simulink model "example9"  (Simulink 6.0)
settings: Solver=ode45  StartTime=0.0  StopTime=100  RelTol=1e-4
undefined symbols (not defined in the file or in its folder): adaptive_passivity, forward_kin_2link, hgoder_2link, parameter_adapt, stateder, Z0, Zhat0
libraries: simulink x1
settings Model: Creator=rhanz  LastModifiedBy=rhanz  ExtModeAutoUpdateStatusClock=off
settings DataIOCC: Refine=2
settings OptimizationCC: InlineInvariantSignals=off

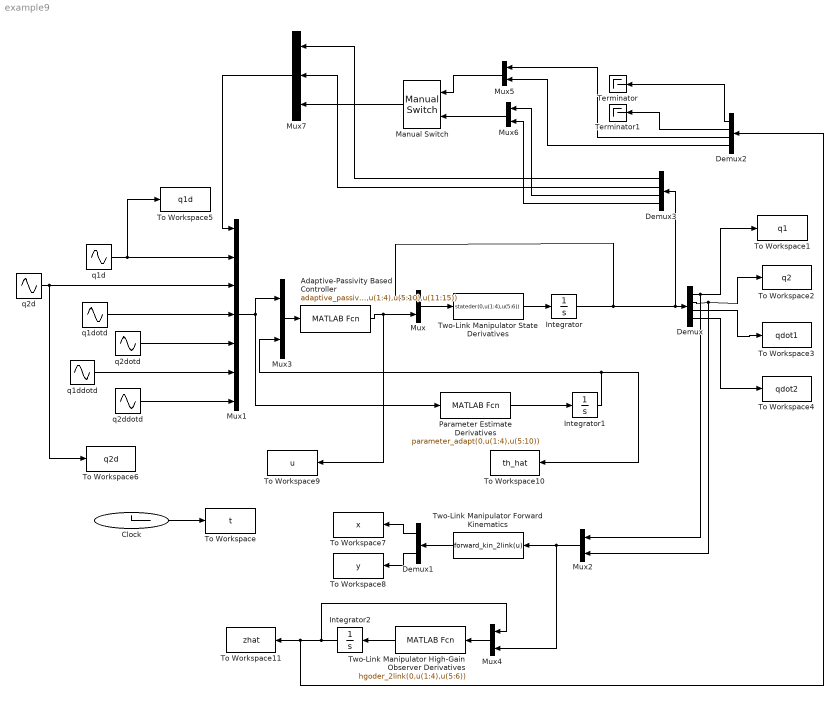
== system example9 ==
  Adaptive-Passivity Based Controller : MATLABFcn  MATLABFcn=adaptive_passivity(0,u(1:4),u(5:10),u(11:15))  OutputDimensions=2
  Clock : Clock
      settings: Decimation=10
  Demux : Demux
  Demux1 : Demux  Orientation=left  Outputs=2
  Demux2 : Demux  Orientation=left
  Demux3 : Demux  Orientation=left
  Integrator : Integrator  InitialCondition=Z0
  Integrator1 : Integrator
  Integrator2 : Integrator  Orientation=left  InitialCondition=Zhat0
  Manual Switch : simulink/Signal Routing/Manual Switch  Orientation=left  sw=1  action=0
  Mux : Mux  Inputs=2
  Mux1 : Mux  Inputs=7
  Mux{2,4..6} (4 alike) : Mux  Orientation=left  Inputs=2
  Mux3 : Mux  Inputs=2
  Mux7 : Mux  Orientation=left  Inputs=3
  Parameter Estimate Derivatives : MATLABFcn  MATLABFcn=parameter_adapt(0,u(1:4),u(5:10))  OutputDimensions=5
  Terminator : Terminator
  Terminator1 : Terminator
  To Workspace : ToWorkspace  VariableName=t  SampleTime=-1  SaveFormat=Array
  To Workspace1 : ToWorkspace  VariableName=q1  SampleTime=-1  SaveFormat=Array
  To Workspace10 : ToWorkspace  VariableName=th_hat  SampleTime=-1  SaveFormat=Array
  To Workspace11 : ToWorkspace  VariableName=zhat  SampleTime=-1  SaveFormat=Array
  To Workspace2 : ToWorkspace  VariableName=q2  SampleTime=-1  SaveFormat=Array
  To Workspace3 : ToWorkspace  VariableName=qdot1  SampleTime=-1  SaveFormat=Array
  To Workspace4 : ToWorkspace  VariableName=qdot2  SampleTime=-1  SaveFormat=Array
  To Workspace5 : ToWorkspace  VariableName=q1d  SampleTime=-1  SaveFormat=Array
  To Workspace6 : ToWorkspace  VariableName=q2d  SampleTime=-1  SaveFormat=Array
  To Workspace7 : ToWorkspace  VariableName=x  SampleTime=-1  SaveFormat=Array
  To Workspace8 : ToWorkspace  VariableName=y  SampleTime=-1  SaveFormat=Array
  To Workspace9 : ToWorkspace  VariableName=u  SampleTime=-1  SaveFormat=Array
  Two-Link Manipulator Forward Kinematics : MATLABFcn  Orientation=left  MATLABFcn=forward_kin_2link(u)  OutputDimensions=2
  Two-Link Manipulator High-Gain Observer Derivatives : MATLABFcn  Orientation=left  MATLABFcn=hgoder_2link(0,u(1:4),u(5:6))
  Two-Link Manipulator State Derivatives : MATLABFcn  MATLABFcn=stateder(0,u(1:4),u(5:6))  OutputDimensions=4
  q1d : Sin  SampleTime=0
  q1ddotd : Sin  Phase=pi  SampleTime=0
  q1dotd : Sin  Phase=pi/2  SampleTime=0
  q2d : Sin  Amplitude=0  Phase=pi/2  SampleTime=0
  q2ddotd : Sin  Amplitude=0  Phase=3*pi/2  SampleTime=0
  q2dotd : Sin  Amplitude=0  Phase=pi  SampleTime=0
  wires:
  Two-Link Manipulator State Derivatives/1 -> Integrator/1
  Integrator/1 -> Mux/1, Demux/1, Demux3/1
  Mux/1 -> Two-Link Manipulator State Derivatives/1
  Clock/1 -> To Workspace/1
  Demux/1 -> To Workspace1/1, Mux2/1
  Demux/2 -> To Workspace2/1, Mux2/2
  Demux/3 -> To Workspace3/1
  Demux/4 -> To Workspace4/1
  Adaptive-Passivity Based Controller/1 -> Mux/2, To Workspace9/1
  q1d/1 -> Mux1/2, To Workspace5/1
  q2d/1 -> Mux1/3, To Workspace6/1
  q1dotd/1 -> Mux1/4
  q2dotd/1 -> Mux1/5
  q1ddotd/1 -> Mux1/6
  q2ddotd/1 -> Mux1/7
  Mux2/1 -> Two-Link Manipulator Forward Kinematics/1, Mux4/2
  Demux1/1 -> To Workspace7/1
  Demux1/2 -> To Workspace8/1
  Two-Link Manipulator Forward Kinematics/1 -> Demux1/1
  Parameter Estimate Derivatives/1 -> Integrator1/1
  Mux1/1 -> Parameter Estimate Derivatives/1, Mux3/1
  Mux3/1 -> Adaptive-Passivity Based Controller/1
  Integrator1/1 -> Mux3/2, To Workspace10/1
  Two-Link Manipulator High-Gain Observer Derivatives/1 -> Integrator2/1
  Mux4/1 -> Two-Link Manipulator High-Gain Observer Derivatives/1
  Integrator2/1 -> Mux4/1, To Workspace11/1, Demux2/1
  Demux2/1 -> Terminator/1
  Demux2/2 -> Terminator1/1
  Demux2/3 -> Mux5/1
  Demux2/4 -> Mux5/2
  Mux5/1 -> Manual Switch/1
  Demux3/3 -> Mux6/1
  Demux3/4 -> Mux6/2
  Mux6/1 -> Manual Switch/2
  Demux3/1 -> Mux7/1
  Demux3/2 -> Mux7/2
  Manual Switch/1 -> Mux7/3
  Mux7/1 -> Mux1/1
